simulink library "simeventssink1"  (Simulink 7.3)
settings: Solver=ode45  SolverMode=SingleTasking  StartTime=0.0  StopTime=10.0  RelTol=1e-3
undefined symbols (not defined in the file or in its folder): des_figposition, des_scope_support, des_support, gcbh
libraries: des_sfun_lib x4, simeventstranslate1 x1
settings Model: Creator=mclune  LastModifiedBy=liw  ExtModeAutoUpdateStatusClock=off
settings Model: ForwardingTableString=|
  | ||__slOldName__||simeventssink1/Discrete Event
  | Scope||__slNewName__||des_test_lib/Discrete Event
  | Scope

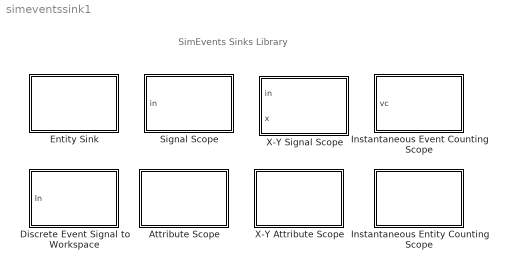
== system simeventssink1 ==
  note: SimEvents Sinks Library
  Attribute Scope : Subsystem  Priority=1  LoadFcn=des_scope_support('desLoadFcn',gcbh)  StartFcn=des_scope_support('desStartFcn',gcbh)  StopFcn=des_scope_support('desStopFcn',gcbh)  mask(Attribute Scope){PlotType=Stair, InputType=Attribute, NumInputs=1, AttributeNameY=Count, XInputOptionSignal=Event time, XInputOptionEntity=Event time, AttributeNameX=Count, EnableEntityOutport=on, XMin=0, XMax=10, XLimitExceededOption=Stretch axis limits, YMin=0, YMax=10, YLimitExceededOption=Stretch axis limits, AxisGrid=on, AxisLegend=off, LineDisables=, LineColors=b, LineStyles=-, LineMarkers=., OpenScopeAtSimStart=on, Title=, YLabel=, XLabel=Time, FigurePosition=des_figposition([5 25 25 25]), AxisZoom=off, DataStoreOption=Limited, DataPointsLimit=10000, StatNumberArrived=Off, ShowCountPlotted=off, ShowToolbar=on}
      mask prompts: PlotType "Plot type:"; InputType "Y value from:"; NumInputs "Number of Y inputs"; AttributeNameY "Y attribute name:"; XInputOptionSignal "X value from:"; XInputOptionEntity "X value from:"; AttributeNameX "X attribute name:"; EnableEntityOutport "Enable entity OUT port"; XMin "Initial X axis lower limit:"; XMax "Initial X axis upper limit:"; XLimitExceededOption "If X value is beyond limit:"; YMin "Initial Y axis lower limit:"; YMax "Initial Y axis upper limit:"; YLimitExceededOption "If Y value is beyond limit:"; AxisGrid "Show grid"; AxisLegend "Legend:"; LineDisables "Line visibility:"; LineColors "Line colors:"; LineStyles "Line styles:"; LineMarkers "Line markers:"; OpenScopeAtSimStart "Open scope at start of simulation"; YLabel "Y label:"; XLabel "X label:"; FigurePosition "Position:"; AxisZoom "Compact display:"; DataStoreOption "Store data when scope is closed:"; DataPointsLimit "Limit data points to:"; StatNumberArrived "Number of entities arrived, #a:"; ShowCountPlotted "Show number of entities"; ShowToolbar "Show Toolbar"
      mask help: Display continuous, stair or stem plot of an attribute versus time or index.
      mask init:
      | des_scopemask2(gcb, 'init','apply')
      settings: CopyFcn=des_scope_support('desCopyFcn',gcbh)  DeleteFcn=des_scope_support('desDeleteFcn',gcbh)  UndoDeleteFcn=des_scope_support('desUndoDeleteFcn',gcbh)  ModelCloseFcn=des_scope_support('desModelCloseFcn',gcbh)  PreSaveFcn=des_scope_support('desPreSaveFcn',gcbh)  PostSaveFcn=des_scope_support('desPostSaveFcn',gcbh)  NameChangeFcn=des_scope_support('desNameChangeFcn',gcbh)  OpenFcn=des_scope_support('desOpenFcn',gcbh)  CloseFcn=des_scope_support('desCloseFcn',gcbh)  ErrorFcn=des_error_redirect
      mask Help: helpview(simeventsbhelp)
      mask StyleString: popup(Stair|Stem|Continuous),popup(Signal|Attribute),edit,edit,popup(Event time|Index|Signal),popup(Event time|Index),edit,checkbox,edit,edit,popup(Stretch axis limits|Keep axis limits unchanged|Shift axis limits),edit,edit,popup(Stretch axis limits|Keep axis limits unchanged|Shift axis limits),checkbox,edit,edit,edit,edit,edit,checkbox,edit,edit,edit,edit,checkbox,popup(Disabled|Unlimited|Limited),edit,popup(Off|On|Upon stop or pause),checkbox,checkbox
      mask CallbackString: des_scopemask2(gcb,'cbPlotType','noapply');|des_scopemask2(gcb,'cbInputType','noapply');|des_scopemask2(gcb,'cbNumInports','noapply');|||des_scopemask2(gcb,'cbXInputOptionEntity','noapply');||des_scopemask2(gcb,'cbEnableEntityOutport','noapply');|||des_scopemask2(gcb,'cbXGrowthOpt','noapply');|||des_scopemask2(gcb,'cbYGrowthOpt','noapply');|||||||||||||des_scopemask2(gcb,'cbDataStoreOption','noapply')||des_scopemask2(gcb,'cbCount','noapply');||
      mask TabNameString: Plotting,Plotting,Plotting,Plotting,Plotting,Plotting,Plotting,Plotting,Axes,Axes,Axes,Axes,Axes,Axes,Axes,Figure,Axes,Axes,Axes,Axes,Plotting,Figure,Figure,Figure,Figure,Figure,Data History,Data History,Statistics,Figure,Figure
      mask Display:
      | image(des_iconLoad('attrScope.jpg'),'center');
      | port_label('LConn',1,'IN');
      | port_label('RConn',1,'OUT');
  Discrete Event Signal to Workspace : Subsystem  mask(Discrete Event Signal to Workspace){VariableName=simout, MaxDataPoints=inf, Decimation=1, SaveFormat=Structure With Time, IsMonitorOnly=off, IsRecordIC=off}
      mask prompts: VariableName "Variable name:"; MaxDataPoints "Limit data points to last:"; SaveFormat "Save format:"; IsMonitorOnly "Is monitor only:"; IsRecordIC "Record initial value"
      mask help:
      | Write discrete event input signal to specific array or structure in base workspace.
      |
      | Data is not available until the simulation is stopped or paused.
      mask init:
      | des_toworkspacemask2(gcb,'init');
      mask Help: helpview(simeventsbhelp)
      mask StyleString: edit,edit,edit,popup(Structure With Time|Structure|Array),checkbox,checkbox
      mask Display: disp(get_param(gcb, 'VariableName'));
  Entity Sink : Subsystem  Priority=1  LoadFcn=des_support('desLoadFcn',gcbh)  StartFcn=des_support('desStartFcn',gcbh)  StopFcn=des_support('desStopFcn',gcbh)  mask(Entity Sink){AvailableForArrivals=on, StatNumberArrived=Off}
      mask prompts: AvailableForArrivals "Input port available for entity arrivals"; StatNumberArrived "Number of entities arrived, #a:"
      mask help: Accept or block entities.
      mask init:
      | des_terminatormask(gcb,'init','apply')
      settings: CopyFcn=des_support('desCopyFcn',gcbh)  DeleteFcn=des_support('desDeleteFcn',gcbh)  UndoDeleteFcn=des_support('desUndoDeleteFcn',gcbh)  ModelCloseFcn=des_support('desModelCloseFcn',gcbh)  PreSaveFcn=des_support('desPreSaveFcn',gcbh)  PostSaveFcn=des_support('desPostSaveFcn',gcbh)  NameChangeFcn=des_support('desNameChangeFcn',gcbh)  CloseFcn=des_support('desCloseFcn',gcbh)  ErrorFcn=des_error_redirect
      mask Help: helpview(simeventsbhelp)
      mask StyleString: checkbox,popup(Off|On|Upon stop or pause)
      mask CallbackString: des_terminatormask(gcb,'cbAvailableForArrivals','noapply');|des_terminatormask(gcb,'cbStatNumberArrived','noapply');
      mask TabNameString: Entity Sink,Entity Sink
      mask Display:
      | image(des_iconLoad('entitySink.jpg'),'center');
      | port_label('LConn',1,'IN');
  Instantaneous Entity Counting Scope : Subsystem  Priority=1  LoadFcn=des_scope_support('desLoadFcn',gcbh)  StartFcn=des_scope_support('desStartFcn',gcbh)  StopFcn=des_scope_support('desStopFcn',gcbh)  mask(Instantaneous Entity Counting Scope){PlotType=Instantaneous entity counting, InputType=Attribute, NumInputs=1, AttributeNameY=Count, XInputOptionSignal=Event time, XInputOptionEntity=Event time, AttributeNameX=Count, EnableEntityOutport=on, XMin=0, XMax=10, XLimitExceededOption=Stretch axis limits, YMin=0, YMax=10, YLimitExceededOption=Stretch axis limits, AxisGrid=on, AxisLegend=off, LineDisables=, LineColors=b, LineStyles=-, LineMarkers=., OpenScopeAtSimStart=on, Title=, YLabel=Number of Entities, XLabel=Time, FigurePosition=des_figposition([5 25 25 25]), AxisZoom=off, DataStoreOption=Limited, DataPointsLimit=10000, StatNumberArrived=Off, ShowCountPlotted=off, ShowToolbar=on}
      mask prompts: PlotType "Plot type:"; InputType "Y value from:"; NumInputs "Number of Y inputs"; AttributeNameY "Y attribute name:"; XInputOptionSignal "X value from:"; XInputOptionEntity "X value from:"; AttributeNameX "X attribute name:"; EnableEntityOutport "Enable entity OUT port"; XMin "Initial X axis lower limit:"; XMax "Initial X axis upper limit:"; XLimitExceededOption "If X value is beyond limit:"; YMin "Initial Y axis lower limit:"; YMax "Initial Y axis upper limit:"; YLimitExceededOption "If Y value is beyond limit:"; AxisGrid "Show grid"; AxisLegend "Legend:"; LineDisables "Line visibility:"; LineColors "Line colors:"; LineStyles "Line styles:"; LineMarkers "Line markers:"; OpenScopeAtSimStart "Open at start of simulation"; YLabel "Y label:"; XLabel "X label:"; FigurePosition "Position:"; AxisZoom "Compact display:"; DataStoreOption "Store data when scope is closed:"; DataPointsLimit "Limit data points to:"; StatNumberArrived "Number of entities arrived, #a:"; ShowCountPlotted "Show number of entities"; ShowToolbar "Show Toolbar"
      mask help: Display entity count versus time.
      mask init:
      | des_scopemask2(gcb, 'init','apply')
      settings: CopyFcn=des_scope_support('desCopyFcn',gcbh)  DeleteFcn=des_scope_support('desDeleteFcn',gcbh)  UndoDeleteFcn=des_scope_support('desUndoDeleteFcn',gcbh)  ModelCloseFcn=des_scope_support('desModelCloseFcn',gcbh)  PreSaveFcn=des_scope_support('desPreSaveFcn',gcbh)  PostSaveFcn=des_scope_support('desPostSaveFcn',gcbh)  NameChangeFcn=des_scope_support('desNameChangeFcn',gcbh)  OpenFcn=des_scope_support('desOpenFcn',gcbh)  CloseFcn=des_scope_support('desCloseFcn',gcbh)  ErrorFcn=des_error_redirect
      mask Help: helpview(simeventsbhelp)
      mask StyleString: popup(Stair|Stem|Continuous|Instantaneous entity counting),popup(Signal|Attribute),edit,edit,popup(Event time|Index|Signal),popup(Event time|Index),edit,checkbox,edit,edit,popup(Stretch axis limits|Keep axis limits unchanged|Shift axis limits),edit,edit,popup(Stretch axis limits|Keep axis limits unchanged|Shift axis limits),checkbox,edit,edit,edit,edit,edit,checkbox,edit,edit,edit,edit,checkbox,popup(Disabled|Unlimited|Limited),edit,popup(Off|On|Upon stop or pause),checkbox,checkbox
      mask CallbackString: des_scopemask2(gcb,'cbPlotType','noapply');|des_scopemask2(gcb,'cbInputType','noapply');|des_scopemask2(gcb,'cbNumInports','noapply');|||des_scopemask2(gcb,'cbXInputOptionEntity','noapply');||des_scopemask2(gcb,'cbEnableEntityOutport','noapply');|||des_scopemask2(gcb,'cbXGrowthOpt','noapply');|||des_scopemask2(gcb,'cbYGrowthOpt','noapply');|||||||||||||des_scopemask2(gcb,'cbDataStoreOption','noapply')||des_scopemask2(gcb,'cbCount','noapply');||
      mask TabNameString: Plotting,Plotting,Plotting,Plotting,Plotting,Plotting,Plotting,Plotting,Axes,Axes,Axes,Axes,Axes,Axes,Axes,Figure,Axes,Axes,Axes,Axes,Plotting,Figure,Figure,Figure,Figure,Figure,Data History,Data History,Figure,Figure,Figure
      mask Display:
      | image(des_iconLoad('countScopeEntity.jpg'),'center');
      | port_label('LConn',1,'IN');
      | port_label('RConn',1,'OUT');
  Instantaneous Event Counting Scope : Subsystem  Priority=1  LoadFcn=des_scope_support('desLoadFcn',gcbh)  StartFcn=des_scope_support('desStartFcn',gcbh)  StopFcn=des_scope_support('desStopFcn',gcbh)  mask(Instantaneous Event Counting Scope){PlotType=Instantaneous event counting, InputType=Signal, NumInputs=1, AttributeNameY=Count, XInputOptionSignal=Event time, XInputOptionEntity=Event time, AttributeNameX=Count, EnableEntityOutport=on, XMin=0, XMax=10, XLimitExceededOption=Stretch axis limits, YMin=0, YMax=10, YLimitExceededOption=Stretch axis limits, AxisGrid=on, AxisLegend=off, LineDisables=, LineColors=b, LineStyles=-, LineMarkers=., OpenScopeAtSimStart=on, Title=, YLabel=Number of Events, XLabel=Time, FigurePosition=des_figposition([5 60 25 25]), AxisZoom=off, DataStoreOption=Limited, DataPointsLimit=10000, StatNumberArrived=Off, ShowCountPlotted=off, PlotPointsUpon=Change in signal from port vc, ChangeType=Rising, ShowToolbar=on}
      mask prompts: PlotType "Plot type:"; InputType "Y value from:"; NumInputs "Number of Y inputs"; AttributeNameY "Y attribute name:"; XInputOptionSignal "X value from:"; XInputOptionEntity "X value from:"; AttributeNameX "X attribute name:"; EnableEntityOutport "Enable entity OUT port"; XMin "Initial X axis lower limit:"; XMax "Initial X axis upper limit:"; XLimitExceededOption "If X value is beyond limit:"; YMin "Initial Y axis lower limit:"; YMax "Initial Y axis upper limit:"; YLimitExceededOption "If Y value is beyond limit:"; AxisGrid "Show grid"; AxisLegend "Legend:"; LineDisables "Line visibility:"; LineColors "Line colors:"; LineStyles "Line styles:"; LineMarkers "Line markers:"; OpenScopeAtSimStart "Open at start of simulation"; YLabel "Y label:"; XLabel "X label:"; FigurePosition "Position:"; AxisZoom "Compact display:"; DataStoreOption "Store data when scope is closed:"; DataPointsLimit "Limit data points to:"; StatNumberArrived "Number of points plotted, #c:"; ShowCountPlotted "Show number of points"; PlotPointsUpon "Plot points upon:"; ChangeType "Type of change in signal value:"; ShowToolbar "Show Toolbar"
      mask help: Display event count plot versus time.
      mask init:
      | des_scopemask_event(gcb, 'init','apply')
      settings: CopyFcn=des_scope_support('desCopyFcn',gcbh)  DeleteFcn=des_scope_support('desDeleteFcn',gcbh)  UndoDeleteFcn=des_scope_support('desUndoDeleteFcn',gcbh)  ModelCloseFcn=des_scope_support('desModelCloseFcn',gcbh)  PreSaveFcn=des_scope_support('desPreSaveFcn',gcbh)  PostSaveFcn=des_scope_support('desPostSaveFcn',gcbh)  NameChangeFcn=des_scope_support('desNameChangeFcn',gcbh)  OpenFcn=des_scope_support('desOpenFcn',gcbh)  CloseFcn=des_scope_support('desCloseFcn',gcbh)  ErrorFcn=des_error_redirect
      mask Help: helpview(simeventsbhelp)
      mask StyleString: popup(Stair|Stem|Continuous|Instantaneous event counting),popup(Signal|Attribute),edit,edit,popup(Event time|Index),popup(Event time|Attribute|Index),edit,checkbox,edit,edit,popup(Stretch axis limits|Keep axis limits unchanged|Shift axis limits),edit,edit,popup(Stretch axis limits|Keep axis limits unchanged|Shift axis limits),checkbox,edit,edit,edit,edit,edit,checkbox,edit,edit,edit,edit,checkbox,popup(Disabled|Unlimited|Limited),edit,popup(Off|On|Upon stop or pause),checkbox,popup(Sample time hit from port ts|Trigger from port tr|Change in signal from port vc|Function call from port fcn),popup(Rising|Falling|Either),checkbox
      mask CallbackString: des_scopemask_event(gcb,'cbPlotType','noapply');|des_scopemask_event(gcb,'cbInputType','noapply');|des_scopemask_event(gcb,'cbNumInports','noapply');||des_scopemask_event(gcb,'cbXInputOptSignal','noapply');|des_scopemask_event(gcb,'cbXInputOptEntity','noapply');||des_scopemask_event(gcb,'cbEnableEntityOutport','noapply');|||des_scopemask_event(gcb,'cbXGrowthOpt','noapply');|||des_scopemask_event(gcb,'cbYGrowthOpt','noapply');|||||||||||||des_scopemask_event(gcb,'cbDataStoreOption','noapply')||des_scopemask_event(gcb,'cbCount','noapply');||des_scopemask_event(gcb,'cbPlotPointsUpon','noapply');||
      mask TabNameString: Plotting,Plotting,Plotting,Plotting,Plotting,Plotting,Plotting,Plotting,Axes,Axes,Axes,Axes,Axes,Axes,Axes,Figure,Axes,Axes,Axes,Axes,Plotting,Figure,Figure,Figure,Figure,Figure,Data History,Data History,Figure,Figure,Plotting,Plotting,Figure
      mask Display:
      | image(des_iconLoad('countScopeEvent.jpg'),'center');
      | port_label('input',1,'vc');
  Signal Scope : Subsystem  Priority=1  LoadFcn=des_scope_support('desLoadFcn',gcbh)  StartFcn=des_scope_support('desStartFcn',gcbh)  StopFcn=des_scope_support('desStopFcn',gcbh)  mask(Signal Scope){PlotType=Stair, InputType=Signal, NumInputs=1, AttributeNameY=Count, XInputOptionSignal=Event time, XInputOptionEntity=Event time, AttributeNameX=Count, EnableEntityOutport=on, XMin=0, XMax=10, XLimitExceededOption=Stretch axis limits, YMin=0, YMax=10, YLimitExceededOption=Stretch axis limits, AxisGrid=on, AxisLegend=off, LineDisables=, LineColors=b, LineStyles=-, LineMarkers=., OpenScopeAtSimStart=on, Title=, YLabel=, XLabel=Time, FigurePosition=des_figposition([5 60 25 25]), AxisZoom=off, DataStoreOption=Limited, DataPointsLimit=10000, StatNumberArrived=Off, ShowCountPlotted=off, ShowToolbar=on}
      mask prompts: PlotType "Plot type:"; InputType "Y value from:"; NumInputs "Number of Y inputs"; AttributeNameY "Y attribute name:"; XInputOptionSignal "X value from:"; XInputOptionEntity "X value from:"; AttributeNameX "X attribute name:"; EnableEntityOutport "Enable entity OUT port"; XMin "Initial X axis lower limit:"; XMax "Initial X axis upper limit:"; XLimitExceededOption "If X value is beyond limit:"; YMin "Initial Y axis lower limit:"; YMax "Initial Y axis upper limit:"; YLimitExceededOption "If Y value is beyond limit:"; AxisGrid "Show grid"; AxisLegend "Legend:"; LineDisables "Line visibility:"; LineColors "Line colors:"; LineStyles "Line styles:"; LineMarkers "Line markers:"; OpenScopeAtSimStart "Open scope at start of simulation"; YLabel "Y label:"; XLabel "X label:"; FigurePosition "Position:"; AxisZoom "Compact display:"; DataStoreOption "Store data when scope is closed:"; DataPointsLimit "Limit data points to:"; StatNumberArrived "Number of points plotted, #c:"; ShowCountPlotted "Show number of points"; ShowToolbar "Show Toolbar"
      mask help: Display continuous, stair, or stem plots of signals versus time or index.
      mask init:
      | des_scopemask2(gcb, 'init','apply')
      settings: CopyFcn=des_scope_support('desCopyFcn',gcbh)  DeleteFcn=des_scope_support('desDeleteFcn',gcbh)  UndoDeleteFcn=des_scope_support('desUndoDeleteFcn',gcbh)  ModelCloseFcn=des_scope_support('desModelCloseFcn',gcbh)  PreSaveFcn=des_scope_support('desPreSaveFcn',gcbh)  PostSaveFcn=des_scope_support('desPostSaveFcn',gcbh)  NameChangeFcn=des_scope_support('desNameChangeFcn',gcbh)  OpenFcn=des_scope_support('desOpenFcn',gcbh)  CloseFcn=des_scope_support('desCloseFcn',gcbh)  ErrorFcn=des_error_redirect
      mask Help: helpview(simeventsbhelp)
      mask StyleString: popup(Stair|Stem|Continuous),popup(Signal|Attribute),edit,edit,popup(Event time|Index),popup(Event time|Attribute|Index),edit,checkbox,edit,edit,popup(Stretch axis limits|Keep axis limits unchanged|Shift axis limits),edit,edit,popup(Stretch axis limits|Keep axis limits unchanged|Shift axis limits),checkbox,edit,edit,edit,edit,edit,checkbox,edit,edit,edit,edit,checkbox,popup(Disabled|Unlimited|Limited),edit,popup(Off|On|Upon stop or pause),checkbox,checkbox
      mask CallbackString: des_scopemask2(gcb,'cbPlotType','noapply');|des_scopemask2(gcb,'cbInputType','noapply');|des_scopemask2(gcb,'cbNumInports','noapply');||des_scopemask2(gcb,'cbXInputOptionSignal','noapply');|des_scopemask2(gcb,'cbXInputOptEntity','noapply');||des_scopemask2(gcb,'cbEnableEntityOutport','noapply');|||des_scopemask2(gcb,'cbXGrowthOpt','noapply');|||des_scopemask2(gcb,'cbYGrowthOpt','noapply');|||||||||||||des_scopemask2(gcb,'cbDataStoreOption','noapply');|des_scopemask2(gcb,'cbDataStoreOption','noapply');|des_scopemask2(gcb,'cbCount','noapply');||
      mask TabNameString: Plotting,Plotting,Plotting,Plotting,Plotting,Plotting,Plotting,Plotting,Axes,Axes,Axes,Axes,Axes,Axes,Axes,Figure,Axes,Axes,Axes,Axes,Plotting,Figure,Figure,Figure,Figure,Figure,Data History,Data History,Statistics,Figure,Figure
      mask Display:
      | image(des_iconLoad('sigScope.jpg'),'center');
      | port_label('input',1,'in');
  X-Y Attribute Scope : Subsystem  Priority=1  LoadFcn=des_scope_support('desLoadFcn',gcbh)  StartFcn=des_scope_support('desStartFcn',gcbh)  StopFcn=des_scope_support('desStopFcn',gcbh)  mask(X-Y Attribute Scope){PlotType=Continuous, InputType=Attribute, NumInputs=1, AttributeNameY=Count, XInputOptionSignal=Event time, XInputOptionEntity=Attribute, AttributeNameX=Count, EnableEntityOutport=on, XMin=0, XMax=10, XLimitExceededOption=Stretch axis limits, YMin=0, YMax=10, YLimitExceededOption=Stretch axis limits, AxisGrid=on, AxisLegend=off, LineDisables=, LineColors=b, LineStyles=-, LineMarkers=., OpenScopeAtSimStart=on, Title=, YLabel=, XLabel=, FigurePosition=des_figposition([5 25 25 25]), AxisZoom=off, DataStoreOption=Limited, DataPointsLimit=10000, StatNumberArrived=Off, ShowCountPlotted=off, ShowToolbar=on}
      mask prompts: PlotType "Plot type:"; InputType "Y value from:"; NumInputs "Number of Y inputs"; AttributeNameY "Y attribute name:"; XInputOptionSignal "X value from:"; XInputOptionEntity "X value from:"; AttributeNameX "X attribute name:"; EnableEntityOutport "Enable entity OUT port"; XMin "Initial X axis lower limit:"; XMax "Initial X axis upper limit:"; XLimitExceededOption "If X value is beyond limit:"; YMin "Initial Y axis lower limit:"; YMax "Initial Y axis upper limit:"; YLimitExceededOption "If Y value is beyond limit:"; AxisGrid "Show grid"; AxisLegend "Legend:"; LineDisables "Line visibility:"; LineColors "Line colors:"; LineStyles "Line styles:"; LineMarkers "Line markers:"; OpenScopeAtSimStart "Open scope at start of simulation"; YLabel "Y label:"; XLabel "X label:"; FigurePosition "Position:"; AxisZoom "Compact display:"; DataStoreOption "Store data when scope is closed:"; DataPointsLimit "Limit data points to:"; StatNumberArrived "Number of entities arrived, #a:"; ShowCountPlotted "Show number of entities"; ShowToolbar "Show Toolbar"
      mask help: Display continuous, stair or stem plot of an attribute versus another attribute.
      mask init:
      | des_scopemask2(gcb, 'init','apply')
      settings: CopyFcn=des_scope_support('desCopyFcn',gcbh)  DeleteFcn=des_scope_support('desDeleteFcn',gcbh)  UndoDeleteFcn=des_scope_support('desUndoDeleteFcn',gcbh)  ModelCloseFcn=des_scope_support('desModelCloseFcn',gcbh)  PreSaveFcn=des_scope_support('desPreSaveFcn',gcbh)  PostSaveFcn=des_scope_support('desPostSaveFcn',gcbh)  NameChangeFcn=des_scope_support('desNameChangeFcn',gcbh)  OpenFcn=des_scope_support('desOpenFcn',gcbh)  CloseFcn=des_scope_support('desCloseFcn',gcbh)  ErrorFcn=des_error_redirect
      mask Help: helpview(simeventsbhelp)
      mask StyleString: popup(Stair|Stem|Continuous),popup(Signal|Attribute),edit,edit,popup(Event time|Index|Signal),popup(Event time|Index|Attribute),edit,checkbox,edit,edit,popup(Stretch axis limits|Keep axis limits unchanged|Shift axis limits),edit,edit,popup(Stretch axis limits|Keep axis limits unchanged|Shift axis limits),checkbox,edit,edit,edit,edit,edit,checkbox,edit,edit,edit,edit,checkbox,popup(Disabled|Unlimited|Limited),edit,popup(Off|On|Upon stop or pause),checkbox,edit
      mask CallbackString: des_scopemask2(gcb,'cbPlotType','noapply');|des_scopemask2(gcb,'cbInputType','noapply');|des_scopemask2(gcb,'cbNumInports','noapply');|||des_scopemask2(gcb,'cbXInputOptionEntity','noapply');||des_scopemask2(gcb,'cbEnableEntityOutport','noapply');|||des_scopemask2(gcb,'cbXGrowthOpt','noapply');|||des_scopemask2(gcb,'cbYGrowthOpt','noapply');|||||||||||||des_scopemask2(gcb,'cbDataStoreOption','noapply')||des_scopemask2(gcb,'cbCount','noapply');||
      mask TabNameString: Plotting,Plotting,Plotting,Plotting,Plotting,Plotting,Plotting,Plotting,Axes,Axes,Axes,Axes,Axes,Axes,Axes,Figure,Axes,Axes,Axes,Axes,Plotting,Figure,Figure,Figure,Figure,Figure,Data History,Data History,Statistics,Figure,Figure
      mask Display:
      | image(des_iconLoad('attrScopeXY.jpg'),'center');
      | port_label('LConn',1,'IN');
      | port_label('RConn',1,'OUT');
  X-Y Signal Scope : Subsystem  Priority=1  LoadFcn=des_scope_support('desLoadFcn',gcbh)  StartFcn=des_scope_support('desStartFcn',gcbh)  StopFcn=des_scope_support('desStopFcn',gcbh)  mask(X-Y Signal Scope){PlotType=Continuous, InputType=Signal, NumInputs=1, AttributeNameY=Count, XInputOptionSignal=Signal, XInputOptionEntity=Event time, AttributeNameX=Count, EnableEntityOutport=on, XMin=0, XMax=10, XLimitExceededOption=Stretch axis limits, YMin=0, YMax=10, YLimitExceededOption=Stretch axis limits, AxisGrid=on, AxisLegend=off, LineDisables=, LineColors=b, LineStyles=-, LineMarkers=., OpenScopeAtSimStart=on, Title=, YLabel=, XLabel=, FigurePosition=des_figposition([5 60 25 25]), AxisZoom=off, DataStoreOption=Limited, DataPointsLimit=10000, StatNumberArrived=Off, ShowCountPlotted=off, ShowToolbar=on}
      mask prompts: PlotType "Plot type:"; InputType "Y value from:"; NumInputs "Number of Y inputs"; AttributeNameY "Y attribute name:"; XInputOptionSignal "X value from:"; XInputOptionEntity "X value from:"; AttributeNameX "X attribute name:"; EnableEntityOutport "Enable entity OUT port"; XMin "Initial X axis lower limit:"; XMax "Initial X axis upper limit:"; XLimitExceededOption "If X value is beyond limit:"; YMin "Initial Y axis lower limit:"; YMax "Initial Y axis upper limit:"; YLimitExceededOption "If Y value is beyond limit:"; AxisGrid "Show grid"; AxisLegend "Legend:"; LineDisables "Line visibility:"; LineColors "Line colors:"; LineStyles "Line styles:"; LineMarkers "Line markers:"; OpenScopeAtSimStart "Open scope at start of simulation"; YLabel "Y label:"; XLabel "X label:"; FigurePosition "Position:"; AxisZoom "Compact display:"; DataStoreOption "Store data when scope is closed:"; DataPointsLimit "Limit data points to:"; StatNumberArrived "Number of points plotted, #c:"; ShowCountPlotted "Show number of points"; ShowToolbar "Show Toolbar"
      mask help: Display continuous, stair, or stem plots of signals versus time or index.
      mask init:
      | des_scopemask2(gcb, 'init','apply')
      settings: CopyFcn=des_scope_support('desCopyFcn',gcbh)  DeleteFcn=des_scope_support('desDeleteFcn',gcbh)  UndoDeleteFcn=des_scope_support('desUndoDeleteFcn',gcbh)  ModelCloseFcn=des_scope_support('desModelCloseFcn',gcbh)  PreSaveFcn=des_scope_support('desPreSaveFcn',gcbh)  PostSaveFcn=des_scope_support('desPostSaveFcn',gcbh)  NameChangeFcn=des_scope_support('desNameChangeFcn',gcbh)  OpenFcn=des_scope_support('desOpenFcn',gcbh)  CloseFcn=des_scope_support('desCloseFcn',gcbh)  ErrorFcn=des_error_redirect
      mask Help: helpview(simeventsbhelp)
      mask StyleString: popup(Stair|Stem|Continuous),popup(Signal|Attribute),edit,edit,popup(Event time|Index|Signal),popup(Event time|Attribute|Index),edit,checkbox,edit,edit,popup(Stretch axis limits|Keep axis limits unchanged|Shift axis limits),edit,edit,popup(Stretch axis limits|Keep axis limits unchanged|Shift axis limits),checkbox,edit,edit,edit,edit,edit,checkbox,edit,edit,edit,edit,checkbox,popup(Disabled|Unlimited|Limited),edit,popup(Off|On|Upon stop or pause),checkbox,checkbox
      mask CallbackString: des_scopemask2(gcb,'cbPlotType','noapply');|des_scopemask2(gcb,'cbInputType','noapply');|des_scopemask2(gcb,'cbNumInports','noapply');||des_scopemask2(gcb,'cbXInputOptionSignal','noapply');|des_scopemask2(gcb,'cbXInputOptEntity','noapply');||des_scopemask2(gcb,'cbEnableEntityOutport','noapply');|||des_scopemask2(gcb,'cbXGrowthOpt','noapply');|||des_scopemask2(gcb,'cbYGrowthOpt','noapply');|||||||||||||des_scopemask2(gcb,'cbDataStoreOption','noapply')||des_scopemask2(gcb,'cbCount','noapply');||
      mask TabNameString: Plotting,Plotting,Plotting,Plotting,Plotting,Plotting,Plotting,Plotting,Axes,Axes,Axes,Axes,Axes,Axes,Axes,Figure,Axes,Axes,Axes,Axes,Plotting,Figure,Figure,Figure,Figure,Figure,Data History,Data History,Statistics,Figure,Figure
      mask Display:
      | image(des_iconLoad('sigScopeXY.jpg'),'center');
      | port_label('input',1,'in');
      | port_label('input',2,'x');

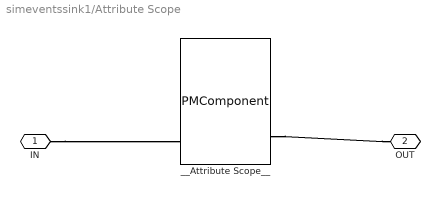
== system simeventssink1/Attribute Scope ==
  __Attribute Scope__ : PMComponent  PhysicalDomain=simevents  SubClassName=DES_SCOPE2  LeftPortType=desPortIn  RightPortType=desPortOut  LConnTagsString=DI|DI|DI  RConnTagsString=DO|DO
      mask Display:
      | port_label('LConn',1,'in');
      | port_label('LConn',2,'x');
      | port_label('LConn',3,'IN');
      | port_label('RConn',1,'#a');
      | port_label('RConn',2,'OUT');
  IN : PMIOPort  Port=1  Side=Left
  OUT : PMIOPort  Orientation=left  Port=2  Side=Right
  connections:
  IN/RConn1 -- __Attribute Scope__/LConn3
  __Attribute Scope__/RConn2 -- OUT/RConn1

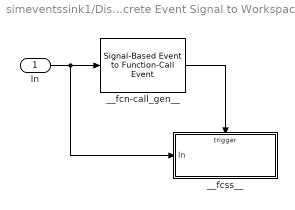
== system simeventssink1/Discrete Event Signal to Workspace ==
  In : Inport
  __fcn-call_gen__ : simeventstranslate1/Signal-Based Event to Function-Call Event  Priority=1  SystemSampleTime=-1  GenerateFunctionCallUpon=Sample time hit from port ts  SignalEdgeOption=Rising  EnableE1Port=off  EnableF2Port=off  EnableE2Port=off  SpecifyEventPriority=off  PriorityFunctionCall=200  FunctionCallDelayFrom=Dialog  DelayFunctionCall=0  StatNumberF1Calls=Off  StatNumberF2Calls=Off  MaskBlockType=TOWKSPC_NO_IC
  __fcss__ : Subsystem  TreatAsAtomicUnit=on
  wires:
  __fcn-call_gen__/1 -> __fcss__/Trigger
  In/1 -> __fcn-call_gen__/1, __fcss__/1(In)

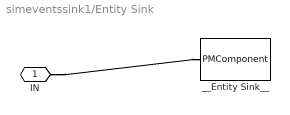
== system simeventssink1/Entity Sink ==
  __Entity Sink__ : PMComponent  PhysicalDomain=simevents  SubClassName=DES_TERMINATOR  LeftPortType=desPortIn  RightPortType=desPortOut  IconImage=body_q.bmp  LConnTagsString=DI  RConnTagsString=DO
      mask Display:
      | port_label('LConn',1,'IN');
      | port_label('RConn',1,'#a');
  IN : PMIOPort  Port=1  Side=Left
  connections:
  IN/RConn1 -- __Entity Sink__/LConn1

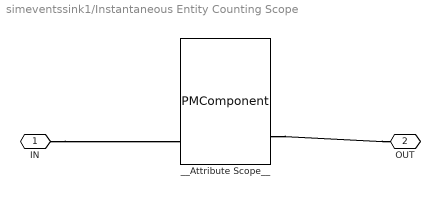
== system simeventssink1/Instantaneous Entity Counting Scope ==
  __Attribute Scope__ : PMComponent  PhysicalDomain=simevents  SubClassName=DES_SCOPE2  LeftPortType=desPortIn  RightPortType=desPortOut  LConnTagsString=DI|DI|DI  RConnTagsString=DO|DO
      mask Display:
      | port_label('LConn',1,'in');
      | port_label('LConn',2,'x');
      | port_label('LConn',3,'IN');
      | port_label('RConn',1,'#a');
      | port_label('RConn',2,'OUT');
  IN : PMIOPort  Port=1  Side=Left
  OUT : PMIOPort  Orientation=left  Port=2  Side=Right
  connections:
  __Attribute Scope__/RConn2 -- OUT/RConn1
  IN/RConn1 -- __Attribute Scope__/LConn3

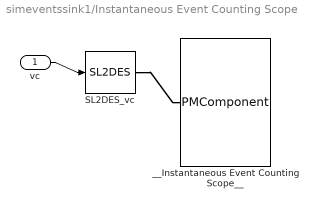
== system simeventssink1/Instantaneous Event Counting Scope ==
  vc : Inport  PortDimensions=1  DataType=double  OutDataType=sfix(16)  OutScaling=2^0  OutDataTypeStr=double
  SL2DES_vc : des_sfun_lib/SL2DES  SystemSampleTime=-1  PortType=desPortOut  PhysicalDomain=simevents  SubClassName=DES_SL2DES  timingControl=Simulink  execIndex=1  trigger=None  filter=0  updateBeforeRead=off  InitValue=0  initToFactVal=off  sampleTime=-1  offsetTime=0  idxBlockMR=0  IsMonitorOnly=on  dimsInfo=1
  __Instantaneous Event Counting Scope__ : PMComponent  PhysicalDomain=simevents  SubClassName=DES_SCOPE_EVENT_COUNTING  LeftPortType=desPortIn  RightPortType=desPortOut  LConnTagsString=DI|DI|DI|DI|DI  RConnTagsString=DO|DO
      mask Display:
      | port_label('LConn',1,'ts');
      | port_label('LConn',2,'tr');
      | port_label('LConn',3,'vc');
      | port_label('LConn',4,'fcn');
      | port_label('LConn',5,'IN');
      | port_label('RConn',1,'#d');
      | port_label('RConn',2,'OUT');
  wires:
  vc/1 -> SL2DES_vc/1
  connections:
  SL2DES_vc/RConn1 -- __Instantaneous Event Counting Scope__/LConn3

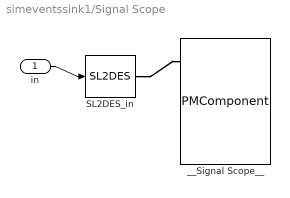
== system simeventssink1/Signal Scope ==
  in : Inport  PortDimensions=1  DataType=double  OutDataType=sfix(16)  OutScaling=2^0  OutDataTypeStr=double
  SL2DES_in : des_sfun_lib/SL2DES  SystemSampleTime=-1  PortType=desPortOut  PhysicalDomain=simevents  SubClassName=DES_SL2DES  timingControl=Simulink  execIndex=1  trigger=None  filter=0  updateBeforeRead=off  InitValue=0  initToFactVal=off  sampleTime=-1  offsetTime=0  idxBlockMR=0  IsMonitorOnly=on  dimsInfo=1
  __Signal Scope__ : PMComponent  PhysicalDomain=simevents  SubClassName=DES_SCOPE2  LeftPortType=desPortIn  RightPortType=desPortOut  LConnTagsString=DI|DI|DI  RConnTagsString=DO|DO
      mask Display:
      | port_label('LConn',1,'in');
      | port_label('LConn',2,'x');
      | port_label('LConn',3,'IN');
      | port_label('RConn',1,'#c');
      | port_label('RConn',2,'OUT');
  wires:
  in/1 -> SL2DES_in/1
  connections:
  SL2DES_in/RConn1 -- __Signal Scope__/LConn1

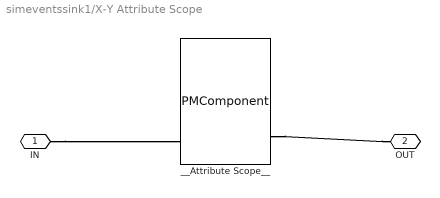
== system simeventssink1/X-Y Attribute Scope ==
  __Attribute Scope__ : PMComponent  PhysicalDomain=simevents  SubClassName=DES_SCOPE2  LeftPortType=desPortIn  RightPortType=desPortOut  LConnTagsString=DI|DI|DI  RConnTagsString=DO|DO
      mask Display:
      | port_label('LConn',1,'in');
      | port_label('LConn',2,'x');
      | port_label('LConn',3,'IN');
      | port_label('RConn',1,'#a');
      | port_label('RConn',2,'OUT');
  IN : PMIOPort  Port=1  Side=Left
  OUT : PMIOPort  Orientation=left  Port=2  Side=Right
  connections:
  __Attribute Scope__/RConn2 -- OUT/RConn1
  IN/RConn1 -- __Attribute Scope__/LConn3

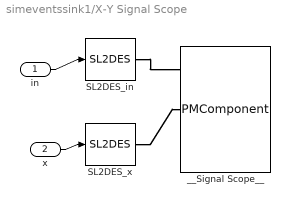
== system simeventssink1/X-Y Signal Scope ==
  in : Inport  PortDimensions=1  DataType=double  OutDataType=sfix(16)  OutScaling=2^0  OutDataTypeStr=double
  x : Inport  Port=2  OutDataType=sfix(16)  OutScaling=2^0
  SL2DES_in : des_sfun_lib/SL2DES  SystemSampleTime=-1  PortType=desPortOut  PhysicalDomain=simevents  SubClassName=DES_SL2DES  timingControl=Simulink  execIndex=1  trigger=None  filter=0  updateBeforeRead=off  InitValue=0  initToFactVal=off  sampleTime=-1  offsetTime=0  idxBlockMR=0  IsMonitorOnly=on  dimsInfo=1
  SL2DES_x : des_sfun_lib/SL2DES  SystemSampleTime=-1  PortType=desPortOut  PhysicalDomain=simevents  SubClassName=DES_SL2DES  timingControl=SimEvents  execIndex=1  trigger=None  filter=0  updateBeforeRead=off  InitValue=0  initToFactVal=off  sampleTime=-1  offsetTime=0  idxBlockMR=0  IsMonitorOnly=off  dimsInfo=1
  __Signal Scope__ : PMComponent  PhysicalDomain=simevents  SubClassName=DES_SCOPE2  LeftPortType=desPortIn  RightPortType=desPortOut  LConnTagsString=DI|DI|DI  RConnTagsString=DO|DO
      mask Display:
      | port_label('LConn',1,'in');
      | port_label('LConn',2,'x');
      | port_label('LConn',3,'IN');
      | port_label('RConn',1,'#c');
      | port_label('RConn',2,'OUT');
  wires:
  x/1 -> SL2DES_x/1
  in/1 -> SL2DES_in/1
  connections:
  SL2DES_x/RConn1 -- __Signal Scope__/LConn2
  SL2DES_in/RConn1 -- __Signal Scope__/LConn1

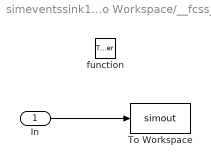
== system simeventssink1/Discrete Event Signal to Workspace/__fcss__ ==
  In : Inport  OutDataType=sfix(16)  OutScaling=2^0
  function : TriggerPort  TriggerType=function-call
  To Workspace : ToWorkspace  VariableName=simout  SampleTime=-1  SaveFormat=Structure With Time
  wires:
  In/1 -> To Workspace/1
